simulink model "simulink_case"  (R2024b)
settings: Solver=ode1  StartTime=0.0  StopTime=T  FixedStep=dt  RelTol=1e-3
values from neighbouring files (symbols this model uses):
  alpha = 0.1    [bench_01_simulink.mat]
settings Model: Creator=aalessan  LastModifiedBy=aalessan

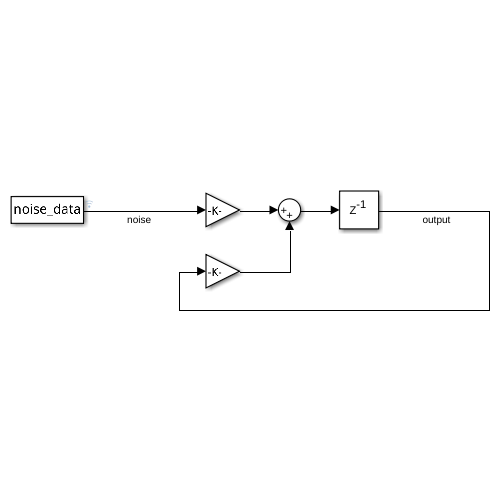
[thumbnail: Simulink's stored preview of the top-level diagram]
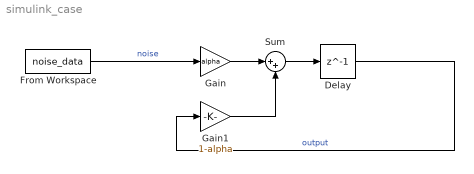
== system simulink_case ==
  Delay : Delay  DelayLength=1
  From Workspace : FromWorkspace  VariableName=noise_data
  Gain : Gain  Gain=alpha
  Gain1 : Gain  Gain=1-alpha
  Sum : Sum  Inputs=|++
  wires:
  Gain/1 -> Sum/1
  Gain1/1 -> Sum/2
  Sum/1 -> Delay/1
  Delay/1 -> Gain1/1  "output"
  From Workspace/1 -> Gain/1  "noise"
